simulink model "tema2ts"  (R2024b)
settings: Solver=VariableStepAuto  StartTime=0.0  StopTime=500  RelTol=1e-3
values from neighbouring files (symbols this model uses):
  kI6 = 3    [tema2.m]
  kI7 = 1    [tema2.m]
  kI8 = -1    [tema2.m]
  kI9 = 0    [tema2.m]
  kR11 = 1    [tema2.m]
  kR12 = 10    [tema2.m]
  kR13 = 0.5    [tema2.m]
  kR14 = 0.1    [tema2.m]
  kR2 = -0.9    [tema2.m]
  kR3 = -0.7    [tema2.m]
  kR4 = -1.5    [tema2.m]
  kR5 = 10    [tema2.m]
  kR6 = 4    [tema2.m]
  kR7 = 1    [tema2.m]
  kR8 = 8    [tema2.m]
  kR9 = 10    [tema2.m]
libraries: slpidlib x2
settings Model: Creator=albertrosca  LastModifiedBy=albertrosca

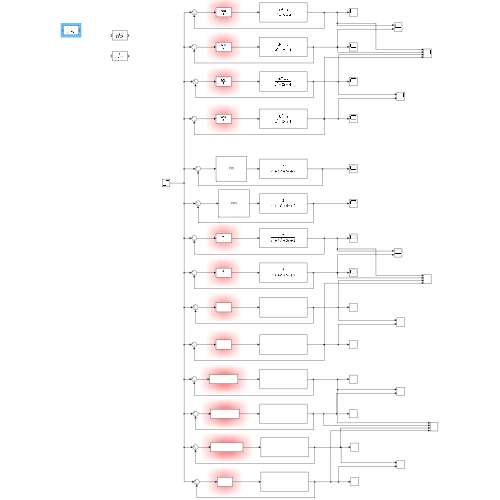
[thumbnail: Simulink's stored preview of the top-level diagram]
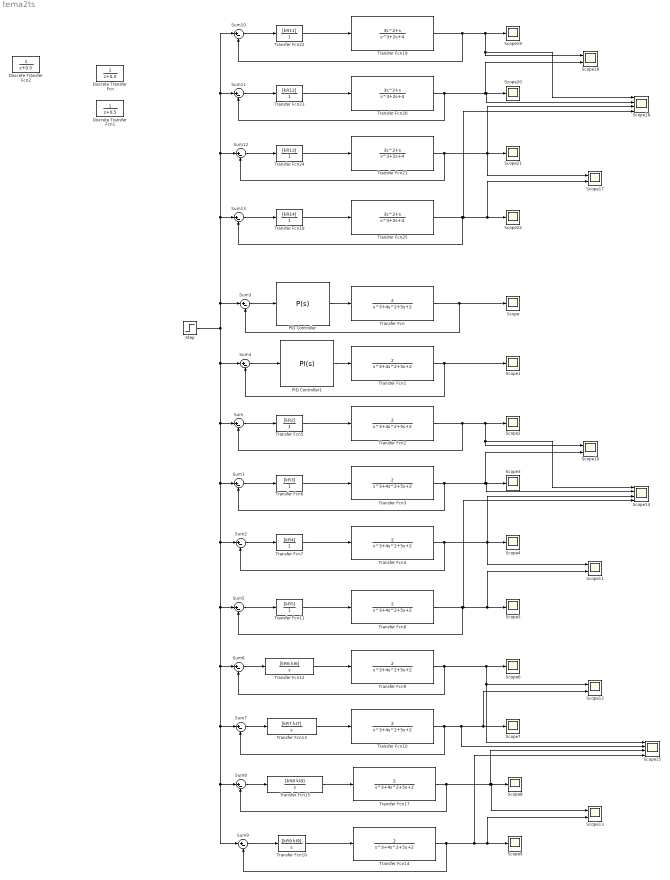
== system tema2ts ==
  Discrete Transfer Fcn : DiscreteTransferFcn  SampleTime=0.005
  Discrete Transfer Fcn1 : DiscreteTransferFcn  a0EqualsOne=on
  Discrete Transfer Fcn2 : DiscreteTransferFcn  SampleTime=0.005
  PID Controller : slpidlib/PID Controller  Controller=P  Form=Parallel  TimeDomain=Continuous-time  UseExternalTs=off  SampleTime=-1  IntegratorMethod=Forward Euler  FilterMethod=Forward Euler  ControllerParametersSource=internal  P=1  I=1  UseKiTs=off  D=0  UseExternalDerivativeSource=off  N=100  UseFilter=on  TunerSelectOption=Transfer Function Based (PID Tuner App)  InitialConditionSource=internal  InitialConditionForIntegrator=0  InitialConditionForFilter=0  DifferentiatorICPrevScaledInput=0  ExternalReset=none  TrackingMode=off  Kt=1  LimitOutput=off  SatLimitsSource=internal  UpperSaturationLimit=inf  LowerSaturationLimit=-inf  LinearizeAsGain=on  AntiWindupMode=none  Kb=1  LimitIntegrator=off  UpperIntegratorSaturationLimit=inf  LowerIntegratorSaturationLimit=-inf  POutMin=[]  POutMax=[]  IOutMin=[]  IOutMax=[]  DOutMin=[]  DOutMax=[]  NOutMin=[]  NOutMax=[]  SumOutMin=[]  SumOutMax=[]  SaturationOutMin=[]  SaturationOutMax=[]  PParamMin=[]  PParamMax=[]  IParamMin=[]  IParamMax=[]  DParamMin=[]  DParamMax=[]  NParamMin=[]  NParamMax=[]  KbParamMin=[]  KbParamMax=[]  KtParamMin=[]  KtParamMax=[]  KbOutMin=[]  KbOutMax=[]  KtOutMin=[]  KtOutMax=[]  IntegratorOutMin=[]  IntegratorOutMax=[]  FilterOutMin=[]  FilterOutMax=[]  SumI1OutMin=[]  SumI1OutMax=[]  SumI2OutMin=[]  SumI2OutMax=[]  SumI3OutMin=[]  SumI3OutMax=[]  SumI4OutMin=[]  SumI4OutMax=[]  SumDOutMin=[]  SumDOutMax=[]  DifferentiatorOutMin=[]  DifferentiatorOutMax=[]  FilterDiffOutCoefMin=[]  FilterDiffOutCoefMax=[]  ReciprocalOutMin=[]  ReciprocalOutMax=[]  SumDenOutMin=[]  SumDenOutMax=[]  SumNumOutMin=[]  SumNumOutMax=[]  DivideOutMin=[]  DivideOutMax=[]  UdiffTsProdOutMin=[]  UdiffTsProdOutMax=[]  NTsProdOutMin=[]  NTsProdOutMax=[]  UintegralTsProdOutMin=[]  UintegralTsProdOutMax=[]  UngainTsProdOutMin=[]  UngainTsProdOutMax=[]  ClampingZeroOutDataTypeStr=Inherit: Inherit via back propagation  ClampingZeroOutMin=[]  ClampingZeroOutMax=[]  FilterDenConstantOutDataTypeStr=Inherit: Inherit via back propagation  FilterDenConstantOutMin=[]  FilterDenConstantOutMax=[]  PCopyOutDataTypeStr=Inherit: Inherit via back propagation  PCopyOutMin=[]  PCopyOutMax=[]  NCopyOutDataTypeStr=Inherit: Inherit via back propagation  NCopyOutMin=[]  NCopyOutMax=[]  IntegratorContinuousStateAttributes=''  IntegratorStateMustResolveToSignalObject=off  IntegratorRTWStateStorageClass=Auto  FilterContinuousStateAttributes=''  FilterStateMustResolveToSignalObject=off  FilterRTWStateStorageClass=Auto  ParallelPVariant=InternalParameters  IdealPVariant=Disabled  IVariant=Disabled  DVariant=Disabled  IntegratorVariant=Disabled  SatVariant=Disabled  AWVariant=Disabled  PCopyVariant=Disabled  TRVariant=Disabled  FdbkBlocksVariant=Forward  IdealPFdbkVariant=Disabled  SatFdbkVariant=Disabled  DerivativeFilterVariant=Disabled  NVariant=Disabled  NCopyVariant=Disabled_SignalSpec  FilterICVariant=Disabled  IntegratorICVariant=Disabled  ExternalResetVariant=Disabled  TRSumVariant=Passthrough  SumFdbkVariant=Disabled  SumVariant=Passthrough_P  TsampFilterVariant=InternalTs  TsampNgainVariant=Passthrough  TsampIntegralVariant=Disabled_SignalSpec  ExternalSaturationOutDataTypeStr=Inherit: Same as second input  DerivativeSourceVariant=Disabled  PreIntVariant=InternalPreInt
  PID Controller1 : slpidlib/PID Controller  Controller=PI  Form=Parallel  TimeDomain=Continuous-time  UseExternalTs=off  SampleTime=-1  IntegratorMethod=Forward Euler  FilterMethod=Forward Euler  ControllerParametersSource=internal  P=1  I=1  UseKiTs=off  D=0  UseExternalDerivativeSource=off  N=100  UseFilter=on  TunerSelectOption=Transfer Function Based (PID Tuner App)  InitialConditionSource=internal  InitialConditionForIntegrator=0  InitialConditionForFilter=0  DifferentiatorICPrevScaledInput=0  ExternalReset=none  TrackingMode=off  Kt=1  LimitOutput=off  SatLimitsSource=internal  UpperSaturationLimit=inf  LowerSaturationLimit=-inf  LinearizeAsGain=on  AntiWindupMode=none  Kb=1  LimitIntegrator=off  UpperIntegratorSaturationLimit=inf  LowerIntegratorSaturationLimit=-inf  POutMin=[]  POutMax=[]  IOutMin=[]  IOutMax=[]  DOutMin=[]  DOutMax=[]  NOutMin=[]  NOutMax=[]  SumOutMin=[]  SumOutMax=[]  SaturationOutMin=[]  SaturationOutMax=[]  PParamMin=[]  PParamMax=[]  IParamMin=[]  IParamMax=[]  DParamMin=[]  DParamMax=[]  NParamMin=[]  NParamMax=[]  KbParamMin=[]  KbParamMax=[]  KtParamMin=[]  KtParamMax=[]  KbOutMin=[]  KbOutMax=[]  KtOutMin=[]  KtOutMax=[]  IntegratorOutMin=[]  IntegratorOutMax=[]  FilterOutMin=[]  FilterOutMax=[]  SumI1OutMin=[]  SumI1OutMax=[]  SumI2OutMin=[]  SumI2OutMax=[]  SumI3OutMin=[]  SumI3OutMax=[]  SumI4OutMin=[]  SumI4OutMax=[]  SumDOutMin=[]  SumDOutMax=[]  DifferentiatorOutMin=[]  DifferentiatorOutMax=[]  FilterDiffOutCoefMin=[]  FilterDiffOutCoefMax=[]  ReciprocalOutMin=[]  ReciprocalOutMax=[]  SumDenOutMin=[]  SumDenOutMax=[]  SumNumOutMin=[]  SumNumOutMax=[]  DivideOutMin=[]  DivideOutMax=[]  UdiffTsProdOutMin=[]  UdiffTsProdOutMax=[]  NTsProdOutMin=[]  NTsProdOutMax=[]  UintegralTsProdOutMin=[]  UintegralTsProdOutMax=[]  UngainTsProdOutMin=[]  UngainTsProdOutMax=[]  ClampingZeroOutDataTypeStr=Inherit: Inherit via back propagation  ClampingZeroOutMin=[]  ClampingZeroOutMax=[]  FilterDenConstantOutDataTypeStr=Inherit: Inherit via back propagation  FilterDenConstantOutMin=[]  FilterDenConstantOutMax=[]  PCopyOutDataTypeStr=Inherit: Inherit via back propagation  PCopyOutMin=[]  PCopyOutMax=[]  NCopyOutDataTypeStr=Inherit: Inherit via back propagation  NCopyOutMin=[]  NCopyOutMax=[]  IntegratorContinuousStateAttributes=''  IntegratorStateMustResolveToSignalObject=off  IntegratorRTWStateStorageClass=Auto  FilterContinuousStateAttributes=''  FilterStateMustResolveToSignalObject=off  FilterRTWStateStorageClass=Auto  ParallelPVariant=InternalParameters  IdealPVariant=Disabled  IVariant=InternalParameters  DVariant=Disabled  IntegratorVariant=Continuous  SatVariant=Disabled  AWVariant=Passthrough  PCopyVariant=Disabled  TRVariant=Disabled  FdbkBlocksVariant=Forward  IdealPFdbkVariant=Disabled  SatFdbkVariant=Disabled  DerivativeFilterVariant=Disabled  NVariant=Disabled  NCopyVariant=Disabled_SignalSpec  FilterICVariant=Disabled  IntegratorICVariant=InternalICs  ExternalResetVariant=Disabled  TRSumVariant=Passthrough  SumFdbkVariant=Disabled  SumVariant=Sum_PI  TsampFilterVariant=InternalTs  TsampNgainVariant=Passthrough  TsampIntegralVariant=Disabled_SignalSpec  ExternalSaturationOutDataTypeStr=Inherit: Same as second input  DerivativeSourceVariant=Disabled  PreIntVariant=InternalPreInt
  Scope{,1..9,19..22} (14 alike) : Scope
  Scope{10..13,16..17} (6 alike) : Scope  NumInputPorts=2
  Scope14 : Scope  NumInputPorts=4
  Scope15 : Scope  NumInputPorts=4
  Scope18 : Scope  NumInputPorts=4
  Step : Step  SampleTime=0
  Sum{,1..13} (14 alike) : Sum  Inputs=|+-
  Transfer Fcn{,1..4,8..10,14,17} (10 alike) : TransferFcn  Numerator=[2]  Denominator=[1 4 5 2]
  Transfer Fcn11 : TransferFcn  Numerator=[kR5]  Denominator=[1]
  Transfer Fcn12 : TransferFcn  Numerator=[kR6 kI6]  Denominator=[1 0]
  Transfer Fcn13 : TransferFcn  Numerator=[kR7 kI7]  Denominator=[1 0]
  Transfer Fcn15 : TransferFcn  Numerator=[kR8 kI8]  Denominator=[1 0]
  Transfer Fcn16 : TransferFcn  Numerator=[kR9 kI9]  Denominator=[1 0]
  Transfer Fcn18 : TransferFcn  Numerator=[kR14]  Denominator=[1]
  Transfer Fcn{19..21,25} (4 alike) : TransferFcn  Numerator=[3 1 0]  Denominator=[1 0 2 4]
  Transfer Fcn22 : TransferFcn  Numerator=[kR11]  Denominator=[1]
  Transfer Fcn23 : TransferFcn  Numerator=[kR12]  Denominator=[1]
  Transfer Fcn24 : TransferFcn  Numerator=[kR13]  Denominator=[1]
  Transfer Fcn5 : TransferFcn  Numerator=[kR2]  Denominator=[1]
  Transfer Fcn6 : TransferFcn  Numerator=[kR3]  Denominator=[1]
  Transfer Fcn7 : TransferFcn  Numerator=[kR4]  Denominator=[1]
  wires:
  PID Controller/1 -> Transfer Fcn/1
  PID Controller1/1 -> Transfer Fcn1/1
  Transfer Fcn1/1 -> Scope1/1, Sum4/2
  Transfer Fcn/1 -> Sum3/2, Scope/1
  Transfer Fcn2/1 -> Sum/2, Scope14/1, Scope10/1, Scope2/1
  Transfer Fcn3/1 -> Scope10/2, Scope14/2, Scope3/1, Sum1/2
  Transfer Fcn4/1 -> Scope11/1, Scope14/3, Scope4/1, Sum2/2
  Transfer Fcn5/1 -> Transfer Fcn2/1
  Transfer Fcn6/1 -> Transfer Fcn3/1
  Transfer Fcn7/1 -> Transfer Fcn4/1
  Sum2/1 -> Transfer Fcn7/1
  Sum1/1 -> Transfer Fcn6/1
  Sum/1 -> Transfer Fcn5/1
  Sum3/1 -> PID Controller/1
  Sum4/1 -> PID Controller1/1
  Transfer Fcn12/1 -> Transfer Fcn9/1
  Transfer Fcn11/1 -> Transfer Fcn8/1
  Transfer Fcn8/1 -> Sum5/2, Scope14/4, Scope11/2, Scope5/1
  Sum6/1 -> Transfer Fcn12/1
  Transfer Fcn10/1 -> Scope15/2, Scope12/2, Scope7/1, Sum7/2
  Sum7/1 -> Transfer Fcn13/1
  Transfer Fcn13/1 -> Transfer Fcn10/1
  Transfer Fcn9/1 -> Scope15/1, Scope12/1, Scope6/1, Sum6/2
  Sum5/1 -> Transfer Fcn11/1
  Transfer Fcn16/1 -> Transfer Fcn14/1
  Transfer Fcn17/1 -> Scope15/3, Scope13/1, Scope8/1, Sum8/2
  Transfer Fcn15/1 -> Transfer Fcn17/1
  Transfer Fcn14/1 -> Scope15/4, Scope13/2, Scope9/1, Sum9/2
  Sum9/1 -> Transfer Fcn16/1
  Sum8/1 -> Transfer Fcn15/1
  Transfer Fcn23/1 -> Transfer Fcn20/1
  Transfer Fcn25/1 -> Sum13/2, Scope18/4, Scope17/2, Scope22/1
  Transfer Fcn24/1 -> Transfer Fcn21/1
  Transfer Fcn22/1 -> Transfer Fcn19/1
  Sum13/1 -> Transfer Fcn18/1
  Transfer Fcn20/1 -> Scope16/2, Scope18/2, Scope20/1, Sum11/2
  Transfer Fcn19/1 -> Sum10/2, Scope18/1, Scope16/1, Scope19/1
  Transfer Fcn21/1 -> Scope17/1, Scope18/3, Scope21/1, Sum12/2
  Sum12/1 -> Transfer Fcn24/1
  Sum10/1 -> Transfer Fcn22/1
  Step/1 -> Sum4/1, Sum7/1, Sum8/1, Sum9/1, Sum6/1, Sum5/1, Sum2/1, Sum1/1, Sum/1, Sum10/1, Sum11/1, Sum12/1, Sum13/1, Sum3/1
  Sum11/1 -> Transfer Fcn23/1
  Transfer Fcn18/1 -> Transfer Fcn25/1
